simulink model "Driving_dynamics_model"  (R2024b)
settings: Solver=VariableStepAuto  StartTime=0.0  StopTime=10.0  RelTol=1e-3
values from neighbouring files (symbols this model uses):
  a = 1.8    [Longitudinal_braking_parameters.m]    (also in Longitudinal_driving_parameters.m)
  A = 1.25    [Longitudinal_braking_parameters.m]    (also in Longitudinal_driving_parameters.m)
  a1 = -1e-5    (= -1e-05)    [Longitudinal_braking_parameters.m]    (also in Longitudinal_driving_parameters.m)
  a2 = 1.25    [Longitudinal_braking_parameters.m]    (also in Longitudinal_driving_parameters.m)
  B = 4.1576    [Longitudinal_braking_parameters.m]    (also in Longitudinal_driving_parameters.m = 5.7507)
  C = 1.7180    (= 1.718)    [Longitudinal_braking_parameters.m]    (also in Longitudinal_driving_parameters.m = 1.2421)
  Cd = 0.6    [Longitudinal_braking_parameters.m]    (also in Longitudinal_driving_parameters.m = 0.4)
  enginemap = [-0.15, 0.23, 0.60, 0.68, 0.8 ... (first row only)    [Longitudinal_driving_parameters.m]
  enginerpm = linspace (1000,15000,15)'    [Longitudinal_driving_parameters.m]
  g = 9.81    [Longitudinal_braking_parameters.m]    (also in Longitudinal_driving_parameters.m)
  h = 0.2    [Longitudinal_braking_parameters.m]    (also in Longitudinal_driving_parameters.m)
  igear = [23.10, 17.64, 13.86, 10.92, 8.82, 7.14, 5.88, 4.33]'    [Longitudinal_driving_parameters.m]
  Iwheel = 0.9    [Longitudinal_braking_parameters.m]    (also in Longitudinal_driving_parameters.m)
  L = 3.5    [Longitudinal_braking_parameters.m]    (also in Longitudinal_driving_parameters.m)
  m = 850    [Longitudinal_braking_parameters.m]    (also in Longitudinal_driving_parameters.m)
  r = 0.375    [Longitudinal_braking_parameters.m]    (also in Longitudinal_driving_parameters.m)
  rho = 1.225    [Longitudinal_braking_parameters.m]    (also in Longitudinal_driving_parameters.m)
  rpm_idling = 1000    [Longitudinal_driving_parameters.m]
  rpm_limit = 15000    [Longitudinal_driving_parameters.m]
  rpm_up = 13500    [Longitudinal_driving_parameters.m]
  Tengmax = 250    [Longitudinal_driving_parameters.m]
  throttlepos = [0, 0.25, 0.5, 0.75, 1]'    [Longitudinal_driving_parameters.m]
settings Model: Creator=jayku  LastModifiedBy=jayku

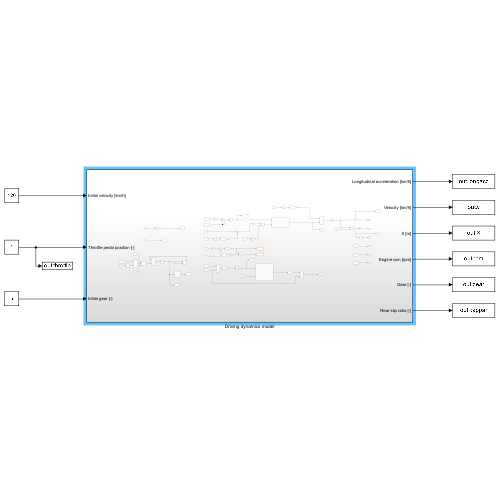
[thumbnail: Simulink's stored preview of the top-level diagram]
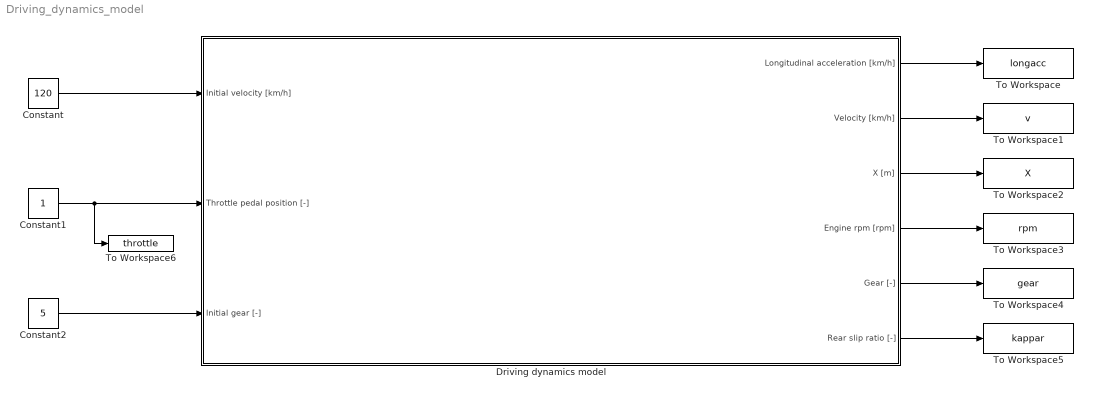
== system Driving_dynamics_model ==
  Constant : Constant  Value=120
  Constant1 : Constant
  Constant2 : Constant  Value=5
  Driving dynamics model : Subsystem
  To Workspace : ToWorkspace  VariableName=longacc  SaveFormat=Timeseries  SampleTime=-1
  To Workspace1 : ToWorkspace  VariableName=v  SaveFormat=Timeseries  SampleTime=-1
  To Workspace2 : ToWorkspace  VariableName=X  SaveFormat=Timeseries  SampleTime=-1
  To Workspace3 : ToWorkspace  VariableName=rpm  SaveFormat=Timeseries  SampleTime=-1
  To Workspace4 : ToWorkspace  VariableName=gear  SaveFormat=Timeseries  SampleTime=-1
  To Workspace5 : ToWorkspace  VariableName=kappar  SaveFormat=Timeseries  SampleTime=-1
  To Workspace6 : ToWorkspace  VariableName=throttle  SaveFormat=Timeseries  SampleTime=-1
  wires:
  Driving dynamics model/1(Longitudinal acceleration [km/h]) -> To Workspace/1
  Driving dynamics model/2(Velocity [km/h]) -> To Workspace1/1
  Driving dynamics model/3(X [m]) -> To Workspace2/1
  Driving dynamics model/4(Engine rpm [rpm]) -> To Workspace3/1
  Driving dynamics model/5(Gear [-]) -> To Workspace4/1
  Driving dynamics model/6(Rear slip ratio [-]) -> To Workspace5/1
  Constant/1 -> Driving dynamics model/1(Initial velocity [km/h])
  Constant2/1 -> Driving dynamics model/3(Initial gear [-])
  Constant1/1 -> To Workspace6/1, Driving dynamics model/2(Throttle pedal position [-])

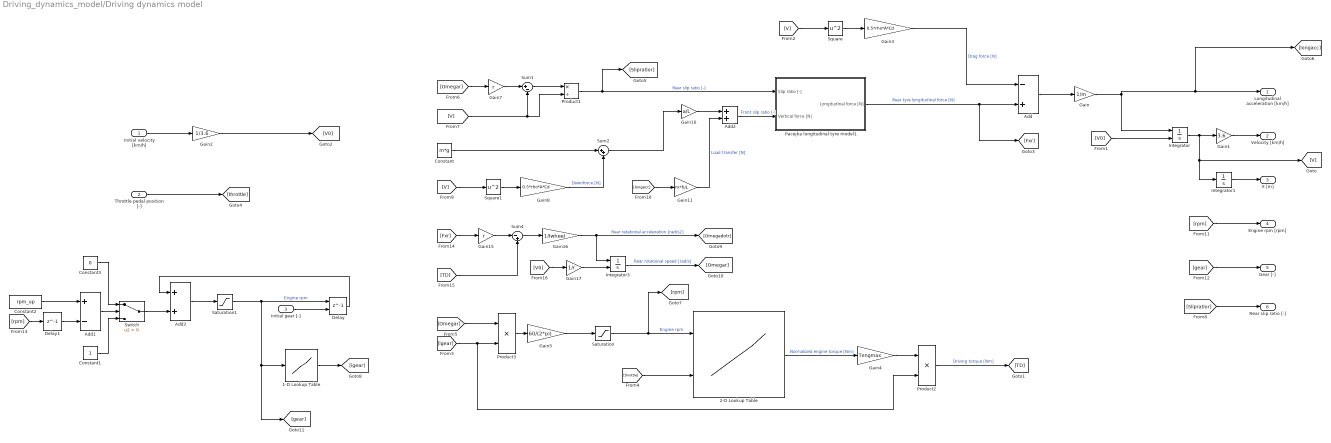
== system Driving_dynamics_model/Driving dynamics model ==
  Initial velocity [km/h] : Inport
  Throttle pedal position [-] : Inport  Port=2
  Initial gear [-] : Inport  Port=3
  1-D Lookup Table : Lookup_n-D  NumberOfTableDimensions=1  BreakpointsForDimension1=[1:8]  Table=igear  InternalRulePriority=Speed  RndMeth=Simplest
  2-D Lookup Table : Lookup_n-D  BreakpointsForDimension1=enginerpm  BreakpointsForDimension2=throttlepos  Table=enginemap  InternalRulePriority=Speed  RndMeth=Simplest
      settings: InputPortMap=u0,u1
  Add : Sum  Inputs=-+
  Add1 : Sum  Inputs=+-
  Add2 : Sum
  Add3 : Sum
  Constant : Constant  Value=m*g
  Constant1 : Constant
  Constant2 : Constant  Value=rpm_up
  Constant3 : Constant  Value=0
  Delay : Delay  DelayLength=1  InitialConditionSource=Input port  InitialCondition=0
      settings: InputPortMap=u0,p4
  Delay1 : Delay  DelayLength=1  InitialCondition=0
  Gain : Gain  Gain=1/m
  Gain1 : Gain  Gain=3.6
  Gain10 : Gain  Gain=a/L
  Gain11 : Gain  Gain=m*h/L
  Gain15 : Gain  Gain=r
  Gain16 : Gain  Gain=1/Iwheel
  Gain17 : Gain  Gain=1/r
  Gain2 : Gain  Gain=1/3.6
  Gain3 : Gain  Gain=0.5*rho*A*Cd
  Gain4 : Gain  Gain=Tengmax
  Gain5 : Gain  Gain=60/(2*pi)
  Gain7 : Gain  Gain=r
  Gain8 : Gain  Gain=0.5*rho*A*Cd
  Integrator : Integrator  InitialConditionSource=external
  Integrator1 : Integrator
  Integrator3 : Integrator  InitialConditionSource=external
  Pacejka longitudinal tyre model1 : Subsystem
  Product1 : Product  Inputs=*/
  Product2 : Product  Inputs=**
  Product3 : Product  Inputs=**
  Saturation : Saturate  UpperLimit=rpm_limit  LowerLimit=rpm_idling
  Saturation1 : Saturate  UpperLimit=length(igear)  LowerLimit=1
  Square : Math  Operator=square
  Square1 : Math  Operator=square
  Sum1 : Sum  Inputs=|+-
  Sum2 : Sum  Inputs=|++
  Sum4 : Sum  Inputs=|-+
  Switch : Switch  Criteria=u2 > Threshold  SaturateOnIntegerOverflow=off  InputSameDT=off
  Longitudinal acceleration [km/h] : Outport
  Velocity [km/h] : Outport  Port=2
  X [m] : Outport  Port=3
  Engine rpm [rpm] : Outport  Port=4
  Gear [-] : Outport  Port=5
  Rear slip ratio [-] : Outport  Port=6
  wires:
  [V0] -> Gain17/1
  [V] -> Square/1
  Add2/1 -> Pacejka longitudinal tyre model1/2(Vertical force [N])  "Front slip ratio [-]"
  Add/1 -> Gain/1
  Gain1/1 -> Velocity [km/h]/1
  Square/1 -> Gain3/1
  [Omegar] -> Gain7/1
  Sum4/1 -> Gain16/1
  Product1/1 -> Pacejka longitudinal tyre model1/1(Slip ratio [-]), [Slipratior]  "Rear slip ratio [-]"
  Sum2/1 -> Gain10/1
  Gain8/1 -> Sum2/2  "Downforce [N]"
  Initial velocity [km/h]/1 -> Gain2/1
  [TD] -> Sum4/2
  Sum1/1 -> Product1/1
  [longacc] -> Gain11/1
  Pacejka longitudinal tyre model1/1(Longitudinal force [N]) -> [Fxr], Add/2  "Rear tyre longitudinal force [N]"
  Gain10/1 -> Add2/1
  Gain2/1 -> [V0]
  Gain7/1 -> Sum1/1
  Integrator3/1 -> [Omegar]  "Rear rotational speed [rad/s]"
  [V0] -> Integrator/2
  Gain/1 -> Integrator/1, [longacc], Longitudinal acceleration [km/h]/1
  [V] -> Product1/2, Sum1/2
  Integrator1/1 -> X [m]/1
  Constant/1 -> Sum2/1
  Gain15/1 -> Sum4/1
  Gain11/1 -> Add2/2  "Load transfer [N]"
  Gain16/1 -> Integrator3/1, [Omegadotr]  "Rear ratational acceleration [rad/s2]"
  Gain3/1 -> Add/1  "Drag force [N]"
  [Slipratior] -> Rear slip ratio [-]/1
  Gain17/1 -> Integrator3/2
  [V] -> Square1/1
  [Fxr] -> Gain15/1
  Integrator/1 -> Integrator1/1, [V], Gain1/1
  Square1/1 -> Gain8/1
  Gain4/1 -> Product2/1
  2-D Lookup Table/1 -> Gain4/1  "Normalized engine torque [Nm]"
  Product2/1 -> [TD]  "Driving torque [Nm]"
  [igear] -> Product3/2, Product2/2
  [throttle] -> 2-D Lookup Table/2
  Throttle pedal position [-]/1 -> [throttle]
  [Omegar] -> Product3/1
  Product3/1 -> Gain5/1
  Gain5/1 -> Saturation/1
  [rpm] -> Engine rpm [rpm]/1
  Saturation/1 -> [rpm], 2-D Lookup Table/1  "Engine rpm"
  Constant2/1 -> Add1/1
  [rpm] -> Delay1/1
  Add1/1 -> Switch/2
  Constant1/1 -> Switch/3
  Constant3/1 -> Switch/1
  Switch/1 -> Add3/2
  Initial gear [-]/1 -> Delay/2
  Add3/1 -> Saturation1/1
  Delay/1 -> Add3/1
  Delay1/1 -> Add1/2
  Saturation1/1 -> Delay/1, 1-D Lookup Table/1, [gear]  "Engine rpm"
  1-D Lookup Table/1 -> [igear]
  [gear] -> Gear [-]/1

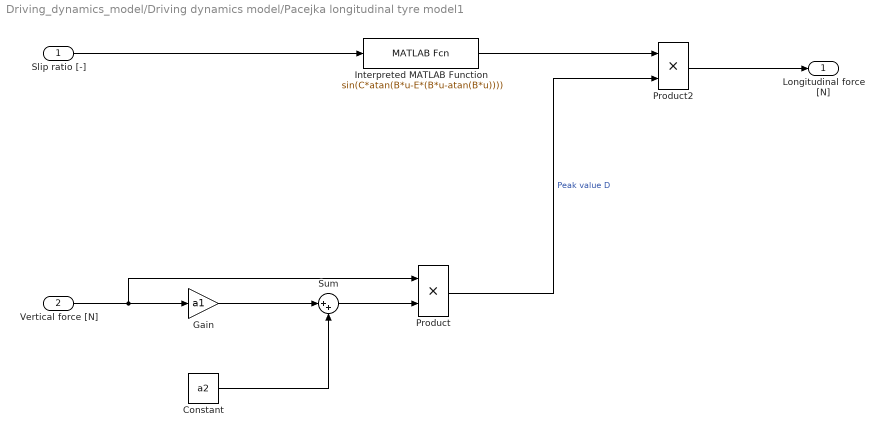
== system Driving_dynamics_model/Driving dynamics model/Pacejka longitudinal tyre model1 ==
  Slip ratio [-] : Inport
  Vertical force [N] : Inport  Port=2
  Constant : Constant  Value=a2
  Gain : Gain  Gain=a1
  Interpreted MATLAB Function : MATLABFcn  MATLABFcn=sin(C*atan(B*u-E*(B*u-atan(B*u))))
  Product : Product
  Product2 : Product
  Sum : Sum  Inputs=|++
  Longitudinal force [N] : Outport
  wires:
  Slip ratio [-]/1 -> Interpreted MATLAB Function/1
  Vertical force [N]/1 -> Product/1, Gain/1
  Gain/1 -> Sum/1
  Constant/1 -> Sum/2
  Sum/1 -> Product/2
  Product/1 -> Product2/2  "Peak value D"
  Interpreted MATLAB Function/1 -> Product2/1
  Product2/1 -> Longitudinal force [N]/1
